simulink model "lab4"  (R2019a)
settings: Solver=VariableStepAuto  StartTime=0.0  StopTime=1000  RelTol=1e-3
libraries: simulink x1
settings Model: Creator=sumli  LastModifiedBy=sumli

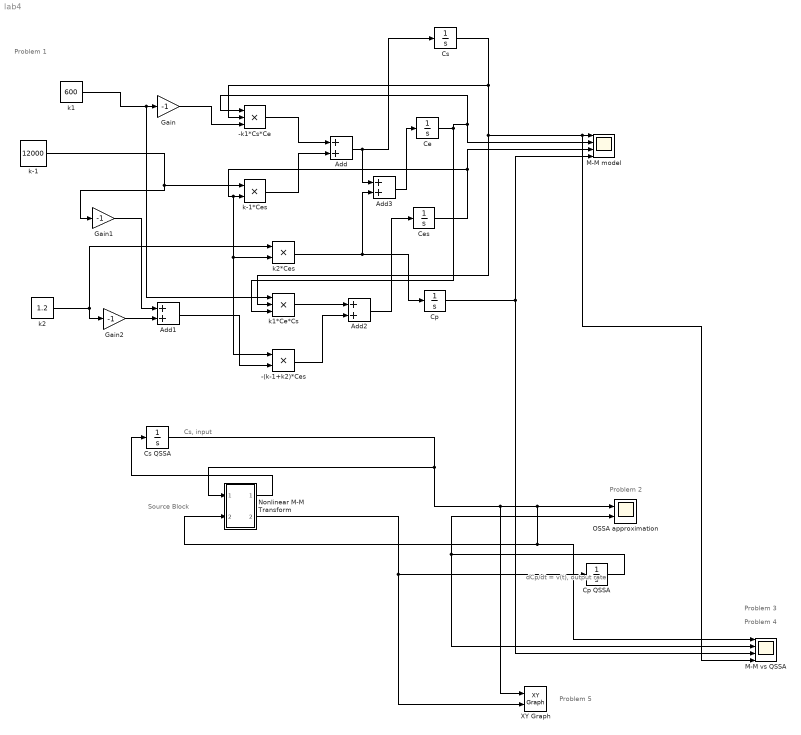
== system lab4 ==
  note: Source Block
  note: dCp/dt = v(t),
      | output rate
  note: Cs, input
  note: Problem 5
  note: Problem 4
  note: Problem 3
  note: Problem 2
  note: Problem 1
  -(k-1+k2)*Ces : Product
  -k1*Cs*Ce : Product  Inputs=3
  Add{,1..3} (4 alike) : Sum
  Ce : Integrator  InitialCondition=1
  Ces : Integrator
  Cp : Integrator
  Cp QSSA : Integrator
  Cs : Integrator  InitialCondition=1
  Cs QSSA : Integrator  InitialCondition=500
  Gain : Gain  Gain=-1
  Gain1 : Gain  Gain=-1
  Gain2 : Gain  Gain=-1
  M-M model : Scope  NumInputPorts=4
  M-M vs QSSA : Scope  NumInputPorts=4
  Nonlinear M-M Transform : Subsystem
  OSSA approximation : Scope  NumInputPorts=2
  XY Graph : simulink/Sinks/XY Graph  xmin=0  xmax=500  ymin=0  ymax=2  st=-1
  k-1 : Constant  Value=12000
  k-1*Ces : Product
  k1 : Constant  Value=600
  k1*Ce*Cs : Product  Inputs=3
  k2 : Constant  Value=1.2
  k2*Ces : Product
  wires:
  k1/1 -> k1*Ce*Cs/1, Gain/1
  k-1/1 -> Gain1/1, k-1*Ces/1
  -k1*Cs*Ce/1 -> Add/1
  k-1*Ces/1 -> Add/2
  Gain/1 -> -k1*Cs*Ce/3
  Add/1 -> Add3/1, Cs/1
  Cs/1 -> M-M vs QSSA/4, M-M model/1, k1*Ce*Cs/2, -k1*Cs*Ce/2
  Ce/1 -> -k1*Cs*Ce/1, M-M model/2, k1*Ce*Cs/3
  Ces/1 -> k2*Ces/2, -(k-1+k2)*Ces/1, k-1*Ces/2, M-M model/3
  k2/1 -> k2*Ces/1, Gain2/1
  Gain2/1 -> Add1/2
  Add1/1 -> -(k-1+k2)*Ces/2
  -(k-1+k2)*Ces/1 -> Add2/2
  k1*Ce*Cs/1 -> Add2/1
  Add2/1 -> Ces/1
  k2*Ces/1 -> Add3/2, Cp/1
  Cp/1 -> M-M vs QSSA/3, M-M model/4
  Gain1/1 -> Add1/1
  Add3/1 -> Ce/1
  Cs QSSA/1 -> XY Graph/1, M-M vs QSSA/1, Nonlinear M-M Transform/2(In2), OSSA approximation/1, Nonlinear M-M Transform/1(In1)
  Cp QSSA/1 -> M-M vs QSSA/2, OSSA approximation/2
  Nonlinear M-M Transform/2(Out2) -> XY Graph/2, Cp QSSA/1
  Nonlinear M-M Transform/1(Out1) -> Cs QSSA/1

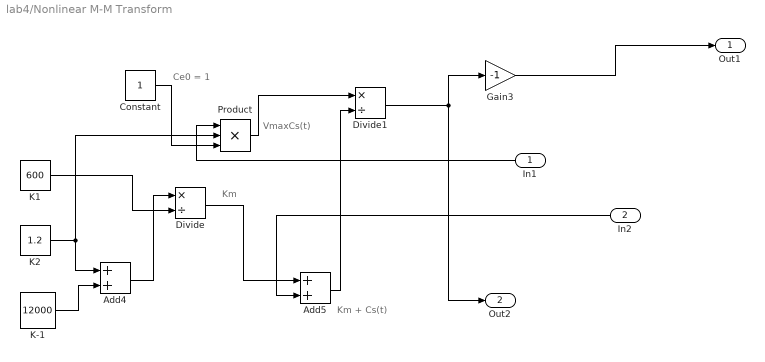
== system lab4/Nonlinear M-M Transform ==
  note: VmaxCs(t)
  note: Ce0 = 1
  note: Km + Cs(t)
  note: Km
  In1 : Inport
  In2 : Inport  Port=2
  Add4 : Sum
  Add5 : Sum
  Constant : Constant
  Divide : Product  Inputs=*/
  Divide1 : Product  Inputs=*/
  Gain3 : Gain  Gain=-1
  K-1 : Constant  Value=12000
  K1 : Constant  Value=600
  "K2 " : Constant  Value=1.2
  Product : Product  Inputs=3
  Out1 : Outport
  Out2 : Outport  Port=2
  wires:
  In2/1 -> Add5/2
  In1/1 -> Product/1
  Add4/1 -> Divide/1
  Divide1/1 -> Out2/1, Gain3/1
  Add5/1 -> Divide1/2
  "K2 "/1 -> Product/2, Add4/1
  K1/1 -> Divide/2
  Divide/1 -> Add5/1
  Constant/1 -> Product/3
  Gain3/1 -> Out1/1
  K-1/1 -> Add4/2
  Product/1 -> Divide1/1
